simulink model "testOctoCtrlRFB"  (R2022b)
settings: Solver=VariableStepAuto  StartTime=0.0  StopTime=40  RelTol=1e-3
undefined symbols (not defined in the file): LF
libraries: instrumentseriallib x3, svdutilitieslib x1
settings Model: Creator=Jovani  LastModifiedBy=Jovani

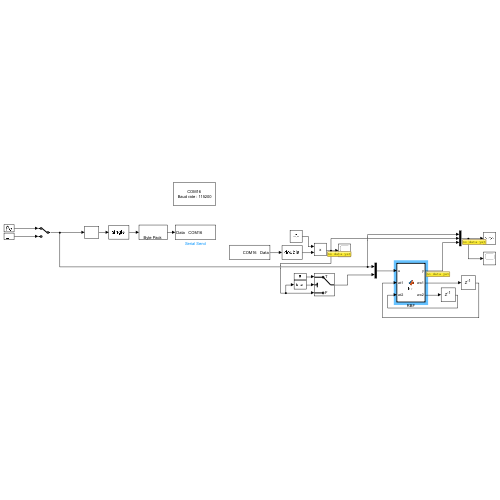
[thumbnail: Simulink's stored preview of the top-level diagram]
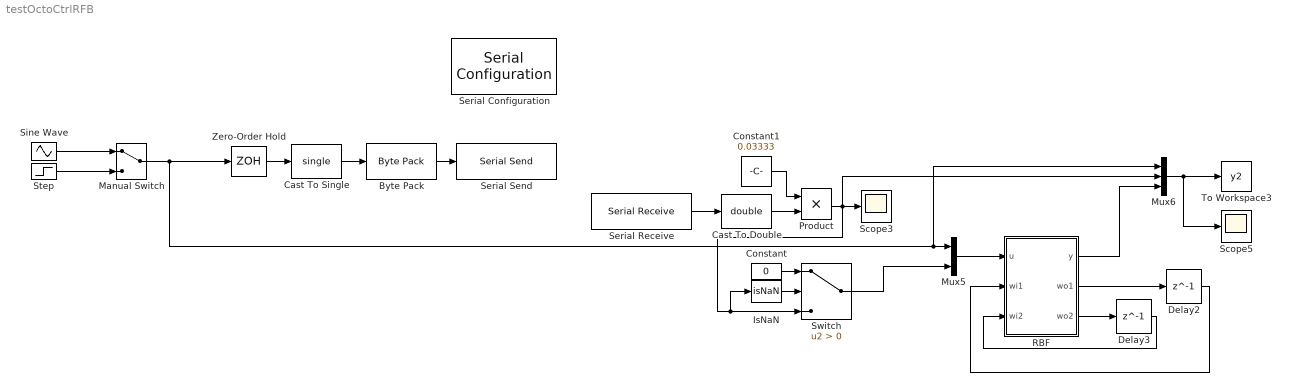
== system testOctoCtrlRFB ==
  Byte Pack : svdutilitieslib/Byte Pack  maskPackedDataType=uint32  datatypes={'single'}  byteAlign=4  blockPlatform=arduinoert
  Cast To Double : DataTypeConversion  OutDataTypeStr=double  SaturateOnIntegerOverflow=off  RndMeth=Floor
  Cast To Single : DataTypeConversion  OutDataTypeStr=single  SaturateOnIntegerOverflow=off  RndMeth=Floor
  Constant : Constant  Value=0
  Constant1 : Constant  Value=0.03333
  Delay2 : Delay  DelayLength=1  InitialCondition=0  SampleTime=0.05
  Delay3 : Delay  DelayLength=1  InitialCondition=0  SampleTime=0.05
  IsNaN : RelationalOperator  Operator=isNaN  OutDataTypeStr=boolean  RndMeth=Simplest  InputSameDT=off
  Manual Switch : ManualSwitch
  Mux5 : Mux  Inputs=2
  Mux6 : Mux  Inputs=3
  Product : Product
  RBF : MATLAB Function  TreatAsAtomicUnit=on
  Scope3 : Scope
  Scope5 : Scope
  Serial Configuration : instrumentseriallib/Serial Configuration  Priority=-200000  PortSel=COM16  Port=COM16  ComPort=COM16  BaudRate=115200  DataBits=8  Parity=none  StopBits=1  ByteOrder=little-endian  FlowControl=none  Timeout=10  SimulateUsing=Interpreted execution  BlockInModel=on  aMode=1
  Serial Receive : instrumentseriallib/Serial Receive  Priority=1  PortSel=COM16  Port=COM16  ComPort=COM16  DataType=single  SaveDataType=uint8  ToggleHeader=on  Header=['A']  ToggleTerminator=on  Terminator=LF ('\n')  CustomTerminator=[]  InputFormat=Column major  ToggleDataSize=on  DataSize=[1 1]  EnableBlockingMode=on  ActionDataUnavailable=Output last received value  ActionWhenDataUnavailable=Output last received value  CustomValue=0  SampleTime=0.05  SimulateUsing=Interpreted execution  BlockInModel=on  aMode=1
  Serial Send : instrumentseriallib/Serial Send  Priority=1  PortSel=COM16  Port=COM16  ComPort=COM16  Header=[]  Terminator=<none>  CustomTerminator=[]  EnableBlockingMode=on  SimulateUsing=Interpreted execution  BlockInModel=on  aMode=1
  Sine Wave : Sin  Frequency=5  SampleTime=0
  Step : Step  SampleTime=0
  Switch : Switch  Criteria=u2 > Threshold  SaturateOnIntegerOverflow=off  InputSameDT=off
  To Workspace3 : ToWorkspace  VariableName=y2  SaveFormat=Timeseries  SampleTime=-1
  Zero-Order Hold : ZeroOrderHold  SampleTime=0.05
  wires:
  Serial Receive/1 -> Cast To Double/1
  Zero-Order Hold/1 -> Cast To Single/1
  Cast To Single/1 -> Byte Pack/1
  Byte Pack/1 -> Serial Send/1
  RBF/2(wo1) -> Delay2/1
  RBF/3(wo2) -> Delay3/1
  Delay3/1 -> RBF/3(wi2)
  Delay2/1 -> RBF/2(wi1)
  Mux6/1 -> Scope5/1, To Workspace3/1
  Mux5/1 -> RBF/1(u)
  Manual Switch/1 -> Mux6/1, Mux5/1, Zero-Order Hold/1
  Sine Wave/1 -> Manual Switch/1
  Step/1 -> Manual Switch/2
  Switch/1 -> Mux5/2
  IsNaN/1 -> Switch/2
  Cast To Double/1 -> Product/2
  Constant/1 -> Switch/1
  RBF/1(y) -> Mux6/3
  Product/1 -> Mux6/2, IsNaN/1, Switch/3, Scope3/1
  Constant1/1 -> Product/1

== matlab function testOctoCtrlRFB/RBF ==
  settings: updateMethod=DISCRETE
  data: u input; y output size=1; wo1 output; wi1 input; wi2 input; wo2 output
function [y,wo1, wo2] = fcn(u, wi1, wi2)

persistent w w_1 w_2 h d_w b ci;
alfa = 0.05;
xite = 0.5;

w_1 = wi1;
w_2 = wi2;

if isempty(w)
        w = rand(5,1);
        b = 5;
        ci = [-5 -2.5 0 2.5 5;
        -10 -5 0 5 10];
        y = u(2);
        wo1 =w;
        wo2 = w_1;
        w_1 = w;
        w_2 = w_1;
        h = zeros(1,5);
        d_w = zeros(1,5);
   return
end

ut = u(1);
ut(isnan(ut)) = 0;


yout = u(2);
 
xi = [ut, yout]';
 
for j=1:1:5
  h(j) = exp(-norm(xi-ci(:,j))^2/(2*b^2));
end

ymout = w'*h';
y = ymout;
 
for j=1:1:5
    d_w(j) = xite*h(j)*(yout-ymout);
end
 
w = w_1 + d_w' +   alfa*(w_1-w_2);

wo1 = w;
wo2 = w_1;
% w_1 = w; 
% w_2 = w_1;
